simulink model "TurnOn_TurnOff_Delay"  (R2025b)
settings: Solver=FixedStepDiscrete  StartTime=0.0  StopTime=10.0  FixedStep=0.1  RelTol=1e-3
libraries: simulink x2
settings Model: Creator=soura  LastModifiedBy=soura

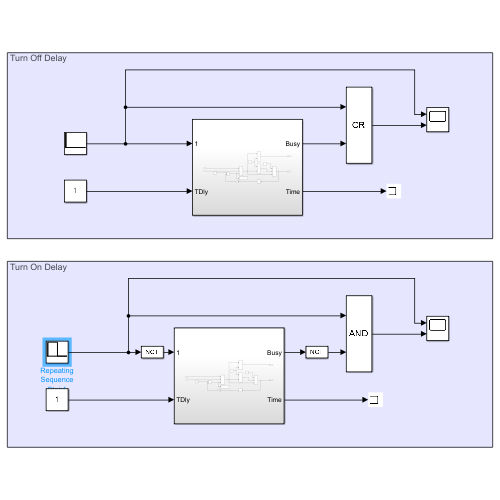
[thumbnail: Simulink's stored preview of the top-level diagram]
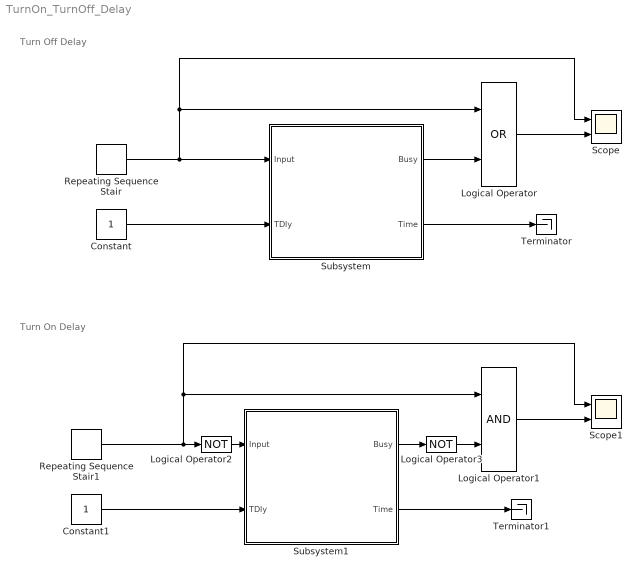
== system TurnOn_TurnOff_Delay ==
  note: Turn Off Delay
  note: Turn On Delay
  Constant : Constant
  Constant1 : Constant
  Logical Operator : Logic  Operator=OR  AllPortsSameDT=off  OutDataTypeStr=boolean
  Logical Operator1 : Logic  AllPortsSameDT=off  OutDataTypeStr=boolean
  Logical Operator2 : Logic  Operator=NOT  AllPortsSameDT=off  OutDataTypeStr=boolean
  Logical Operator3 : Logic  Operator=NOT  AllPortsSameDT=off  OutDataTypeStr=boolean
  Repeating Sequence Stair : simulink/Sources/Repeating Sequence Stair  OutValues=[0 1 0 0 0 0 0 0 0 0 0 0 0 0 0 0 0 0 0 0 0 0 0 0 0 0 0 0 0 0 0 0].'  tsamp=-1  OutMin=[]  OutMax=[]  OutDataTypeStr=double  OutputDataTypeScalingMode=double  OutDataType=fixdt(0,8)  ConRadixGroup=Best Precision: Vector-wise  OutScaling=2^-12
  Repeating Sequence Stair1 : simulink/Sources/Repeating Sequence Stair  OutValues=[0 1 1 1 1 1 1 1 1 1 1 1 1 1 0 0 0 0 0 0 0 0 0 0 0 0 0].'  tsamp=-1  OutMin=[]  OutMax=[]  OutDataTypeStr=double  OutputDataTypeScalingMode=double  OutDataType=fixdt(0,8)  ConRadixGroup=Best Precision: Vector-wise  OutScaling=2^-12
  Scope : Scope  NumInputPorts=2
      settings: ActiveDisplayYMinimum=-1  ActiveDisplayYMaximum=1
  Scope1 : Scope  NumInputPorts=2
      settings: ActiveDisplayYMinimum=-0.12499999999999997  ActiveDisplayYMaximum=1.125
  Subsystem : Subsystem
  Subsystem1 : Subsystem
  Terminator : Terminator
  Terminator1 : Terminator
  wires:
  Constant/1 -> Subsystem/2(TDly)
  Repeating Sequence Stair/1 -> Subsystem/1(Input), Logical Operator/1, Scope/1
  Subsystem/2(Time) -> Terminator/1
  Subsystem/1(Busy) -> Logical Operator/2
  Logical Operator/1 -> Scope/2
  Logical Operator1/1 -> Scope1/2
  Subsystem1/2(Time) -> Terminator1/1
  Constant1/1 -> Subsystem1/2(TDly)
  Repeating Sequence Stair1/1 -> Logical Operator2/1, Logical Operator1/1, Scope1/1
  Subsystem1/1(Busy) -> Logical Operator3/1
  Logical Operator3/1 -> Logical Operator1/2
  Logical Operator2/1 -> Subsystem1/1(Input)

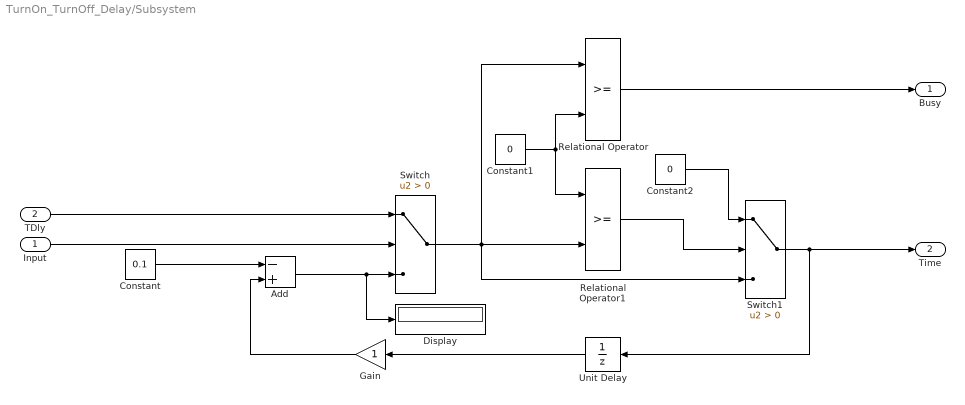
== system TurnOn_TurnOff_Delay/Subsystem ==
  Input : Inport
  TDly : Inport  Port=2
  Add : Sum  Inputs=-+
  Constant : Constant  Value=0.1  OutDataTypeStr=fixdt(1,8,0.1,0)
  Constant1 : Constant  Value=0
  Constant2 : Constant  Value=0
  Display : Display
  Gain : Gain  OutDataTypeStr=fixdt(1,8,0.1,0)
  Relational Operator : RelationalOperator  OutDataTypeStr=boolean  RndMeth=Simplest  InputSameDT=off
  Relational Operator1 : RelationalOperator  OutDataTypeStr=boolean  RndMeth=Simplest  InputSameDT=off
  Switch : Switch  Criteria=u2 > Threshold  SaturateOnIntegerOverflow=off  InputSameDT=off
  Switch1 : Switch  Criteria=u2 > Threshold  OutDataTypeStr=single  SaturateOnIntegerOverflow=off  InputSameDT=off
  Unit Delay : UnitDelay  SampleTime=-1  HasFrameUpgradeWarning=on
  Busy : Outport
  Time : Outport  Port=2
  wires:
  Switch/1 -> Relational Operator1/2, Switch1/3, Relational Operator/1
  Relational Operator1/1 -> Switch1/2
  Switch1/1 -> Time/1, Unit Delay/1
  Input/1 -> Switch/2
  Add/1 -> Display/1, Switch/3
  Constant1/1 -> Relational Operator1/1, Relational Operator/2
  Relational Operator/1 -> Busy/1
  Constant/1 -> Add/1
  Constant2/1 -> Switch1/1
  TDly/1 -> Switch/1
  Unit Delay/1 -> Gain/1
  Gain/1 -> Add/2

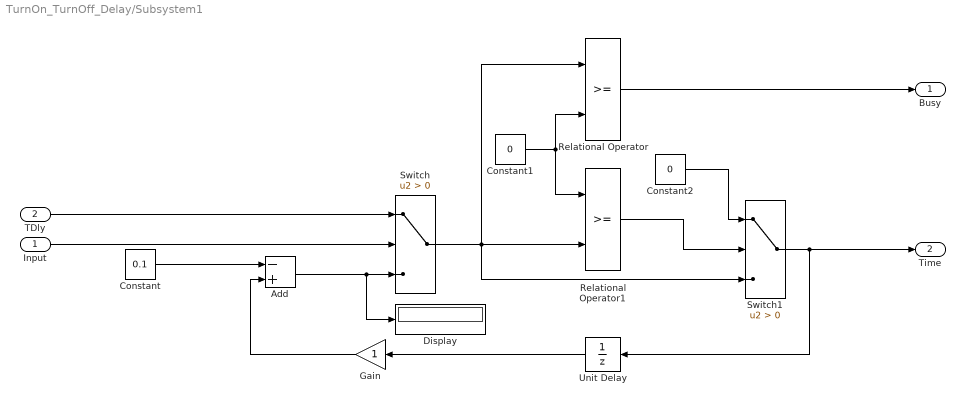
== system TurnOn_TurnOff_Delay/Subsystem1 ==
  Input : Inport
  TDly : Inport  Port=2
  Add : Sum  Inputs=-+
  Constant : Constant  Value=0.1  OutDataTypeStr=fixdt(1,8,0.1,0)
  Constant1 : Constant  Value=0
  Constant2 : Constant  Value=0
  Display : Display
  Gain : Gain  OutDataTypeStr=fixdt(1,8,0.1,0)
  Relational Operator : RelationalOperator  OutDataTypeStr=boolean  RndMeth=Simplest  InputSameDT=off
  Relational Operator1 : RelationalOperator  OutDataTypeStr=boolean  RndMeth=Simplest  InputSameDT=off
  Switch : Switch  Criteria=u2 > Threshold  SaturateOnIntegerOverflow=off  InputSameDT=off
  Switch1 : Switch  Criteria=u2 > Threshold  OutDataTypeStr=single  SaturateOnIntegerOverflow=off  InputSameDT=off
  Unit Delay : UnitDelay  SampleTime=-1  HasFrameUpgradeWarning=on
  Busy : Outport
  Time : Outport  Port=2
  wires:
  Gain/1 -> Add/2
  Unit Delay/1 -> Gain/1
  TDly/1 -> Switch/1
  Constant2/1 -> Switch1/1
  Constant/1 -> Add/1
  Relational Operator/1 -> Busy/1
  Constant1/1 -> Relational Operator/2, Relational Operator1/1
  Add/1 -> Switch/3, Display/1
  Input/1 -> Switch/2
  Switch1/1 -> Unit Delay/1, Time/1
  Relational Operator1/1 -> Switch1/2
  Switch/1 -> Relational Operator/1, Switch1/3, Relational Operator1/2
